simulink model "Sinus"  (R2015a)
settings: Solver=ode45  SolverMode=SingleTasking  StartTime=0.0  StopTime=600  MaxStep=1e-3  RelTol=1e-3
values from neighbouring files (symbols this model uses):
  A = double(subs(A_sym, params, vals))    [Main.m]
  A_phi = 0    [Main.m]
  A_psi = 1    [Main.m]
  A_theta = 0    [Main.m]
  A_z = 0    [Main.m]
  B = double(subs(B_sym, params, vals))    [Main.m]
  b = 2.92e-6    (= 2.92e-06)    [Main.m]
  C = [1 0 0 0 0 0 0 0; 0 0 1 0 0 0 0 0; 0 0 0 1 0 0 0 0; 0 0 0 0 1 0 0 0]    [Main.m]
  d = 1.12e-7    (= 1.12e-07)    [Main.m]
  eul_0 = [0.1; -0.1; 0.1]    [Main.m]
  g = 9.81    [Main.m]
  I = [I_xx I_xy I_xz ... (first row only)    [Main.m]
  k3 = k_bar(:,1:8)    [Main.m]
  k4 = k_bar(:,9:12)    [Main.m]
  L = 0.2    [Main.m]
  L_observer = (place(A',C',p_2))'    [Main.m]
  m = 0.5    [Main.m]
  pm_0 = [0.01; -0.01; 0.01]    [Main.m]
  r_0 = [0; 0; 0.1]    [Main.m]
  rdot_0 = [0; 0; 0.01]    [Main.m]
  tau = 1    [Main.m]
libraries: simulink_extras x6, aerolibutil x1, aerolibtransform2 x1
settings Model: CovMetricSettings=dwe  CovHtmlReporting=off  covSaveCumulativeToWorkspaceVar=off  CovSaveSingleToWorkspaceVar=off  CovExternalEMLEnable=on  Creator=Masoud Nateghi  LastModifiedBy=soren
settings DataIOCC: LimitDataPoints=off  SaveFormat=StructureWithTime  ReturnWorkspaceOutputs=on
settings DebuggingCC: SFUnexpectedBacktrackingDiag=error  SFNoUnconditionalDefaultTransitionDiag=error
settings HardwareCC: ProdBitPerPointer=64  ProdLargestAtomicFloat=Float  ProdIntDivRoundTo=Zero  ProdEndianess=LittleEndian  ProdHWDeviceType=Specified
settings ModelReferenceCC: PropagateSignalLabelsOutOfModel=on
settings SFSimCC: SimUseLocalCustomCode=on
settings RTWCC: RTWUseLocalCustomCode=on
settings GRTTargetCC: TargetLangStandard=C99 (ISO)

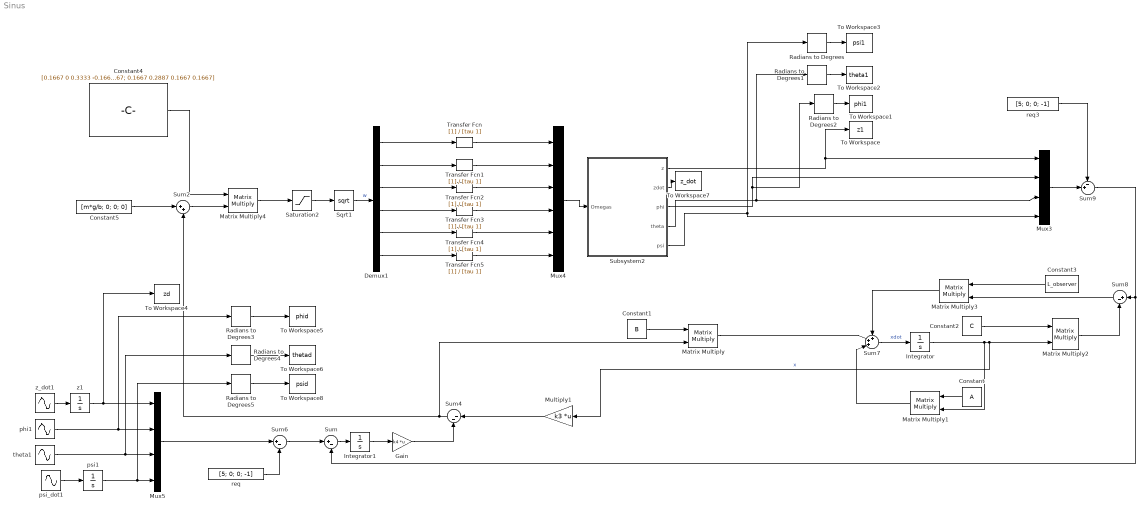
== system Sinus ==
  Constant : Constant  Value=A  VectorParams1D=off
  Constant1 : Constant  Value=B  VectorParams1D=off
  Constant2 : Constant  Value=C  VectorParams1D=off
  Constant3 : Constant  Value=L_observer  VectorParams1D=off
  Constant4 : Constant  Value=[0.1667 0 0.3333 -0.1667; 0.1667 -0.2887 0.1667 0.1667; 0.1667 -0.2887 -0.1667 -0.1667; 0.1667 0 -0.3333 0.1667; 0.1667 0.2887 -0.1667 -0.1667; 0.1667 0.2887 0.1667 0.1667]
  Constant5 : Constant  Value=[m*g/b; 0; 0; 0]
  Demux1 : Demux  Outputs=6
  Gain : Gain  Gain=k4  Multiplication=Matrix(K*u)
  Integrator : Integrator  InitialCondition=[1; 0; -0.1; 0.1; 1.5; 0; 0; 0]
  Integrator1 : Integrator  InitialCondition=[0;0;0;0]
  Matrix Multiply{,1..4} (5 alike) : Product  Multiplication=Matrix(*)
  Multiply1 : Gain  Gain=k3  Multiplication=Matrix(K*u)
  Mux3 : Mux
  Mux4 : Mux  Inputs=6
  Mux5 : Mux
  Radians to Degrees{,1..5} (6 alike) : simulink_extras/Transformations/Radians to Degrees
  Saturation2 : Saturate  UpperLimit=inf  LowerLimit=0
  Sqrt1 : Sqrt  SaturateOnIntegerOverflow=on
  Subsystem2 : Subsystem
  Sum : Sum  Inputs=|+-
  Sum2 : Sum  Inputs=|++
  Sum4 : Sum  Inputs=|--
  Sum6 : Sum  Inputs=|+-
  Sum7 : Sum  Inputs=+++|
  Sum8 : Sum  Inputs=|+-
  Sum9 : Sum  Inputs=-+|
  To Workspace : ToWorkspace  VariableName=z1  SampleTime=-1
      settings: Save2DSignal=2-D array (concatenate along first dimension)
  To Workspace1 : ToWorkspace  VariableName=phi1  SampleTime=-1
      settings: Save2DSignal=2-D array (concatenate along first dimension)
  To Workspace2 : ToWorkspace  VariableName=theta1  SampleTime=-1
      settings: Save2DSignal=2-D array (concatenate along first dimension)
  To Workspace3 : ToWorkspace  VariableName=psi1  SampleTime=-1
      settings: Save2DSignal=2-D array (concatenate along first dimension)
  To Workspace4 : ToWorkspace  VariableName=zd  SampleTime=-1
      settings: Save2DSignal=2-D array (concatenate along first dimension)
  To Workspace5 : ToWorkspace  VariableName=phid  SampleTime=-1
      settings: Save2DSignal=2-D array (concatenate along first dimension)
  To Workspace6 : ToWorkspace  VariableName=thetad  SampleTime=-1
      settings: Save2DSignal=2-D array (concatenate along first dimension)
  To Workspace7 : ToWorkspace  VariableName=z_dot  SampleTime=-1
      settings: Save2DSignal=2-D array (concatenate along first dimension)
  To Workspace8 : ToWorkspace  VariableName=psid  SampleTime=-1
      settings: Save2DSignal=2-D array (concatenate along first dimension)
  Transfer Fcn{,1..5} (6 alike) : TransferFcn  Denominator=[tau 1]
  phi1 : Sin  Amplitude=A_phi  Frequency=1/20  SampleTime=0
  psi1 : Integrator
  psi_dot1 : Sin  Amplitude=A_psi  Frequency=1/20  SampleTime=0
  req : Constant  Value=[5; 0; 0; -1]
  req3 : Constant  Value=[5; 0; 0; -1]
  theta1 : Sin  Amplitude=A_theta  Frequency=1/20  SampleTime=0
  z1 : Integrator
  z_dot1 : Sin  Amplitude=A_z  Frequency=1/20  SampleTime=0
  wires:
  phi1/1 -> Radians to Degrees3/1, Mux5/2
  Matrix Multiply4/1 -> Saturation2/1
  Transfer Fcn3/1 -> Mux4/4
  Matrix Multiply1/1 -> Sum7/3
  Radians to Degrees/1 -> To Workspace3/1
  Matrix Multiply2/1 -> Sum8/2
  theta1/1 -> Radians to Degrees4/1, Mux5/3
  Sum9/1 -> Sum/2, Sum8/1
  Demux1/6 -> Transfer Fcn5/1
  Transfer Fcn5/1 -> Mux4/6
  Subsystem2/2(zdot) -> To Workspace7/1
  Constant2/1 -> Matrix Multiply2/1
  Sum7/1 -> Integrator/1  "xdot"
  z_dot1/1 -> z1/1
  Matrix Multiply3/1 -> Sum7/1
  Transfer Fcn/1 -> Mux4/1
  Radians to Degrees2/1 -> To Workspace1/1
  Subsystem2/1(z) -> To Workspace/1, Mux3/1
  Demux1/2 -> Transfer Fcn1/1
  Sum4/1 -> Matrix Multiply/2, Sum2/2
  Integrator/1 -> Multiply1/1, Matrix Multiply2/2, Matrix Multiply1/2  "x"
  Subsystem2/3(phi) -> Mux3/2, Radians to Degrees2/1
  Sum8/1 -> Matrix Multiply3/2
  Mux3/1 -> Sum9/2
  Constant3/1 -> Matrix Multiply3/1
  Sqrt1/1 -> Demux1/1  "w"
  Constant1/1 -> Matrix Multiply/1
  Sum2/1 -> Matrix Multiply4/2
  Transfer Fcn4/1 -> Mux4/5
  psi1/1 -> Radians to Degrees5/1, Mux5/4
  Demux1/5 -> Transfer Fcn4/1
  req/1 -> Sum6/2
  Transfer Fcn2/1 -> Mux4/3
  Demux1/4 -> Transfer Fcn3/1
  Mux4/1 -> Subsystem2/1(Omegas)
  Constant/1 -> Matrix Multiply1/1
  Constant4/1 -> Matrix Multiply4/1
  Demux1/3 -> Transfer Fcn2/1
  Transfer Fcn1/1 -> Mux4/2
  Constant5/1 -> Sum2/1
  Saturation2/1 -> Sqrt1/1
  Subsystem2/5(psi) -> Mux3/4, Radians to Degrees/1
  Matrix Multiply/1 -> Sum7/2
  req3/1 -> Sum9/1
  Mux5/1 -> Sum6/1
  Subsystem2/4(theta) -> Radians to Degrees1/1, Mux3/3
  psi_dot1/1 -> psi1/1
  Demux1/1 -> Transfer Fcn/1
  Multiply1/1 -> Sum4/1
  Radians to Degrees1/1 -> To Workspace2/1
  Radians to Degrees3/1 -> To Workspace5/1
  Radians to Degrees5/1 -> To Workspace8/1
  Radians to Degrees4/1 -> To Workspace6/1
  z1/1 -> To Workspace4/1, Mux5/1
  Sum6/1 -> Sum/1
  Sum/1 -> Integrator1/1
  Gain/1 -> Sum4/2
  Integrator1/1 -> Gain/1

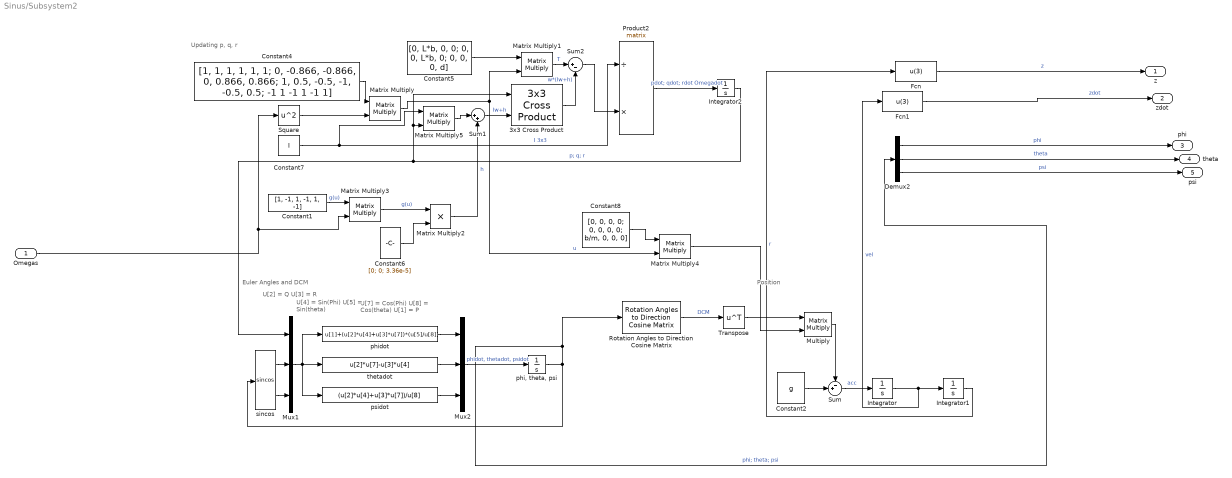
== system Sinus/Subsystem2 ==
  note: Euler Angles and DCM
  note: Updating p, q, r
  note: Position
  note: U[7] = Cos(Phi)
      | U[8] = Cos(theta)
      | U[1] = P
  note: U[2] = Q
      | U[3] = R
  note: U[4] = Sin(Phi)
      | U[5] = Sin(theta)
  Omegas : Inport
  3x3 Cross Product : aerolibutil/3x3 Cross Product
  Constant1 : Constant  Value=[1, -1, 1, -1, 1, -1]  VectorParams1D=off
  Constant2 : Constant  Value=g  VectorParams1D=off
  Constant4 : Constant  Value=[1, 1, 1, 1, 1, 1; 0, -0.866, -0.866, 0, 0.866, 0.866; 1, 0.5, -0.5, -1, -0.5, 0.5; -1 1 -1 1 -1 1]
  Constant5 : Constant  Value=[0, L*b, 0, 0; 0, 0, L*b, 0; 0, 0, 0, d]
  Constant6 : Constant  Value=[0; 0; 3.36e-5]  VectorParams1D=off
  Constant7 : Constant  Value=I
  Constant8 : Constant  Value=[0, 0, 0, 0; 0, 0, 0, 0; b/m, 0, 0, 0]
  Demux2 : Demux  Outputs=3
  Fcn : Fcn  Expr=u(3)
  Fcn1 : Fcn  Expr=u(3)
  Integrator : Integrator  InitialCondition=rdot_0
  Integrator1 : Integrator  InitialCondition=r_0
  Integrator2 : Integrator  InitialCondition=pm_0
  Matrix Multiply{,1,3..5} (5 alike) : Product  Multiplication=Matrix(*)
  Matrix Multiply2 : Product
  Multiply : Product  Multiplication=Matrix(*)
  Mux1 : Mux  Inputs=[3 3 3]
  Mux2 : Mux  Inputs=3
  Product2 : Product  Inputs=/*  Multiplication=Matrix(*)  SaturateOnIntegerOverflow=on  OutDataTypeStr=Inherit: Same as first input
  Rotation Angles to Direction Cosine Matrix : aerolibtransform2/Rotation Angles to Direction Cosine Matrix  rotationOrder=XYZ
  Square : Math  Operator=square  SaturateOnIntegerOverflow=on
  Sum : Sum  Inputs=-+|
  Sum1 : Sum  Inputs=|++  SaturateOnIntegerOverflow=on
  Sum2 : Sum  Inputs=|+-  SaturateOnIntegerOverflow=on
  Transpose : Math  Operator=transpose  SaturateOnIntegerOverflow=on
  "phi, theta, psi" : Integrator  InitialCondition=eul_0  WrapState=on
  phidot : Fcn  Expr=u[1]+(u[2]*u[4]+u[3]*u[7])*(u[5]/u[8])
  psidot : Fcn  Expr=(u[2]*u[4]+u[3]*u[7])/u[8]
  sincos : Trigonometry  Operator=sincos
  thetadot : Fcn  Expr=u[2]*u[7]-u[3]*u[4]
  z : Outport
  zdot : Outport  Port=2
  phi : Outport  Port=3
  theta : Outport  Port=4
  psi : Outport  Port=5
  wires:
  "phi, theta, psi"/1 -> Rotation Angles to Direction Cosine Matrix/1, Demux2/1, sincos/1  "phi; theta; psi"
  Transpose/1 -> Multiply/1
  Constant5/1 -> Matrix Multiply1/1
  psidot/1 -> Mux2/3
  Integrator2/1 -> Mux1/1, 3x3 Cross Product/1, Matrix Multiply5/2  "p; q; r"
  Square/1 -> Matrix Multiply/2
  Constant7/1 -> Matrix Multiply5/1, Product2/1  "I 3x3"
  Constant1/1 -> Matrix Multiply3/1  "g(u)"
  Integrator1/1 -> Fcn/1  "r"
  Matrix Multiply5/1 -> Sum1/1
  Matrix Multiply1/1 -> Sum2/1  "T"
  Matrix Multiply3/1 -> Matrix Multiply2/1  "g(u)"
  Constant6/1 -> Matrix Multiply2/2
  Mux1/1 -> psidot/1, phidot/1, thetadot/1
  Constant4/1 -> Matrix Multiply/1
  sincos/2 -> Mux1/3
  Mux2/1 -> "phi, theta, psi"/1  "phidot, thetadot, psidot"
  Constant8/1 -> Matrix Multiply4/1
  Constant2/1 -> Sum/2
  3x3 Cross Product/1 -> Sum2/2  "w*(Iw+h)"
  Matrix Multiply2/1 -> Sum1/2  "h"
  Multiply/1 -> Sum/1
  Sum1/1 -> 3x3 Cross Product/2  "Iw+h"
  Sum/1 -> Integrator/1  "acc"
  Matrix Multiply4/1 -> Multiply/2
  Integrator/1 -> Fcn1/1, Integrator1/1  "vel"
  sincos/1 -> Mux1/2
  Fcn/1 -> z/1  "z"
  Omegas/1 -> Square/1, Matrix Multiply3/2
  Matrix Multiply/1 -> Matrix Multiply1/2, Matrix Multiply4/2  "u"
  Fcn1/1 -> zdot/1  "zdot"
  Demux2/3 -> psi/1  "psi"
  phidot/1 -> Mux2/1
  Product2/1 -> Integrator2/1  "pdot; qdot; rdot Omegadot"
  Demux2/2 -> theta/1  "theta"
  thetadot/1 -> Mux2/2
  Rotation Angles to Direction Cosine Matrix/1 -> Transpose/1  "DCM"
  Sum2/1 -> Product2/2
  Demux2/1 -> phi/1  "phi"
